simulink model "VVI_good"  (R2020a)
settings: Solver=FixedStepAuto  StartTime=0.0  StopTime=10.0  FixedStep=1e-3  RelTol=1e-3  EnableMultiTasking=on
undefined symbols (not defined in the file): D1, D10, D12, D13, D2, D3, D5, D7, D9, PTA1, PTA2, PTB9, PTC17, PTC3, PTC4, PTD0, PTD1, PTD3
libraries: frdmk64flib x9
settings Model: ExtModeTrigDuration=5  Creator=hinda  LastModifiedBy=hinda
settings OptimizationCC: EnhancedBackFolding=on  PassReuseOutputArgsAs=Individual arguments  ZeroExternalMemoryAtStartup=off  ZeroInternalMemoryAtStartup=off  MaxStackSize=64  OptimizeBlockOrder=speed  DifferentSizesBufferReuse=on  OptimizationCustomize=off  EfficientTunableParamExpr=on
settings DebuggingCC: ParameterTunabilityLossMsg=error
settings HardwareCC: ProdBitPerPointer=32  ProdBitPerSizeT=32  ProdBitPerPtrDiffT=32  ProdLargestAtomicInteger=Long  ProdLargestAtomicFloat=Double  ProdWordSize=32  ProdHWDeviceType=ARM Compatible->ARM Cortex
settings SFSimCC: MATLABDynamicMemAlloc=off
settings RTWCC: SystemTargetFile=ert.tlc  HardwareBoard=NXP FRDM-K64F  TemplateMakefile=ert_default_tmf  Toolchain=GNU Tools for ARM Embedded Processors
settings CodeAppCC: ForceParamTrailComments=on  IgnoreCustomStorageClasses=off  OperatorAnnotations=on  SimulinkDataObjDesc=on  SFDataObjDesc=on  InsertBlockDesc=on

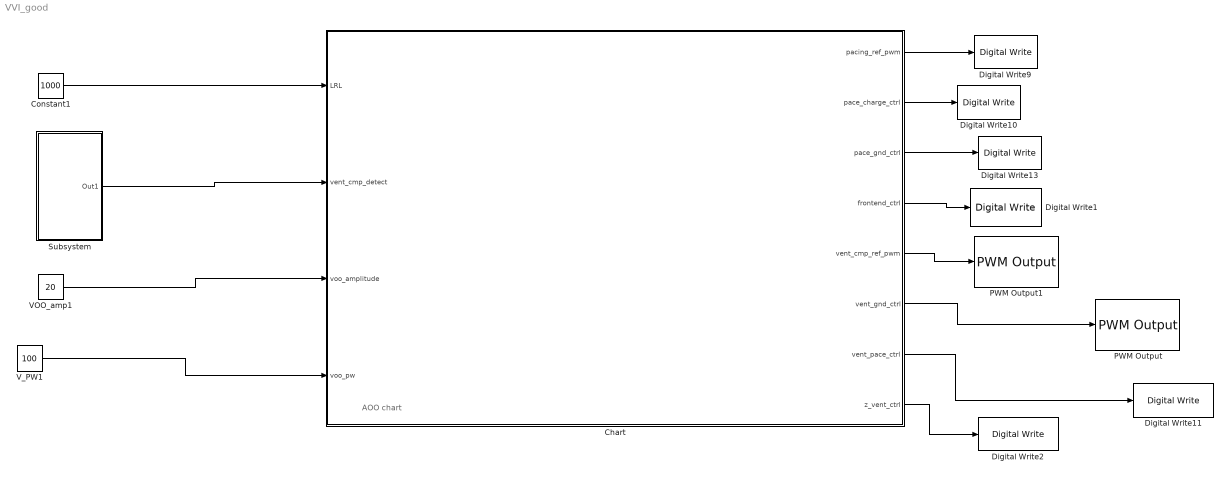
== system VVI_good ==
  note: AOO chart
  Chart : Stateflow chart  TreatAsAtomicUnit=on
  Constant1 : Constant  Value=1000
  Digital Write1 : frdmk64flib/Digital Write  Whichpin=PTD1 (D13)
  Digital Write10 : frdmk64flib/Digital Write  Whichpin=PTB9 (D2)
  Digital Write11 : frdmk64flib/Digital Write  Whichpin=PTC4 (D9)
  Digital Write13 : frdmk64flib/Digital Write  Whichpin=PTD0 (D10)
  Digital Write2 : frdmk64flib/Digital Write  Whichpin=PTC3 (D7)
  Digital Write9 : frdmk64flib/Digital Write  Whichpin=PTA2 (D5)
  PWM Output : frdmk64flib/PWM Output  Whichpin=PTD3 (D12)  InitialFrequency=2000  InitialDutyCycle=0
  PWM Output1 : frdmk64flib/PWM Output  Whichpin=PTA1 (D3)  InitialFrequency=2000  InitialDutyCycle=0
  Subsystem : Subsystem
  VOO_amp1 : Constant  Value=20
  V_PW1 : Constant  Value=100
  wires:
  Subsystem/1(Out1) -> Chart/2(vent_cmp_detect)
  Chart/1(pacing_ref_pwm) -> Digital Write9/1
  Chart/3(pace_gnd_ctrl) -> Digital Write13/1
  Chart/2(pace_charge_ctrl) -> Digital Write10/1
  Chart/4(frontend_ctrl) -> Digital Write1/1
  V_PW1/1 -> Chart/4(voo_pw)
  Constant1/1 -> Chart/1(LRL)
  VOO_amp1/1 -> Chart/3(voo_amplitude)
  Chart/6(vent_gnd_ctrl) -> PWM Output/1
  Chart/7(vent_pace_ctrl) -> Digital Write11/1
  Chart/8(z_vent_ctrl) -> Digital Write2/1
  Chart/5(vent_cmp_ref_pwm) -> PWM Output1/1

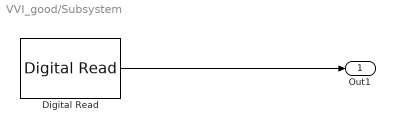
== system VVI_good/Subsystem ==
  Digital Read : frdmk64flib/Digital Read  Whichpin=PTC17 (D1)  SampleTime=-1
  Out1 : Outport
  wires:
  Digital Read/1 -> Out1/1

== stateflow chart VVI_good/Chart ==
  state charging
    entry:
    %charging C22
    %discharging C21
    vent_pace_ctrl = 0; %do not want c22 to discharge
    pacing_ref_pwm = voo_amplitude; %send in signal
    pace_charge_ctrl = 1;
    pace_gnd_ctrl = 0; %discharges C21
    vent_gnd_ctrl = 1; %1 when discharging through atrium
    %average threshold amplitude is 80
    z_vent_ctrl = 0; %connects impedance circuit to atrium ring electrode output is at z_signal pin
    %sensing
    frontend_ctrl = 1;
    vent_cmp_ref_pwm = 80; %send in threshold signal, if heart is less then we will send signal
  state pacing
    entry:
    %charging C21
    %discharging C22
    vent_gnd_ctrl = 0;
    vent_pace_ctrl = 1;
    z_vent_ctrl = 0;
    pace_charge_ctrl = 0;
    pace_gnd_ctrl = 1;
    pacing_ref_pwm = voo_amplitude;
    frontend_ctrl = 0;
  (junction 61) -> charging [order 1] : [vent_cmp_detect == 1]
  (default) -> charging
  charging -> (junction 61)
  (junction 61) -> pacing [order 2] : after(LRL-voo_pw, msec)[vent_cmp_detect==0]
  pacing -> charging : [after(voo_pw, msec)]
  data: LRL input; pacing_ref_pwm output; pace_charge_ctrl output; pace_gnd_ctrl output; frontend_ctrl output; vent_cmp_detect input; voo_amplitude input; voo_pw input; vent_cmp_ref_pwm output; vent_gnd_ctrl output; vent_pace_ctrl output; z_vent_ctrl output
